simulink model "Biped_Model1"  (R2019a)
settings: Solver=VariableStepAuto  StartTime=0.0  StopTime=Time(end)  FixedStep=.001  EnableMultiTasking=on
PreLoadFcn:
  | YBT_HomeDir = pwd;
  | 
  | % Code to use copy within this repository
  | addpath([YBT_HomeDir filesep 'Libraries' filesep 'CFL_Libs']);
  | startup_Contact_Forces
  | 
  | cd(YBT_HomeDir)
  | addpath(YBT_HomeDir);
  | addpath([YBT_HomeDir filesep 'Libraries']);
  | addpath([YBT_HomeDir filesep 'Images']);
  | 
  | Robot_Parameters
model workspace: external: MATLAB File C:\Users\nozaripo\Desktop\BipedalWalking_Simulink_ModelnData\Robot_Parameters.m (data not in the file)
values from neighbouring files (symbols this model uses):
  ankle_servo_kd = 4    [Robot_Parameters.m]
  ankle_servo_ki = 0    [Robot_Parameters.m]
  ankle_servo_kp = 70    [Robot_Parameters.m]
  ankle_to_midLow = 19    [Robot_Parameters.m]
  contact_damping = 50    [Robot_Parameters.m]
  contact_point_radius = 0.005    [Robot_Parameters.m]
  contact_stiffness = 90311    [Robot_Parameters.m]
  deriv_filter_coeff = 50    [Robot_Parameters.m]
  foot_mass = 1    [Robot_Parameters.m]
  height_plane = 0.1    [Robot_Parameters.m]
  hip_servo_kd = 30    [Robot_Parameters.m]
  hip_servo_ki = 0    [Robot_Parameters.m]
  hip_servo_kp = 300    [Robot_Parameters.m]
  init = -joint_angles(1,:)    [Script_Data.m]
  init_vel = -vel(1,:)    [Script_Data.m]
  joint_angles = joint_angles(:,end:-1:1)    [Script_Data.m]
  joint_damping = 0    [Robot_Parameters.m]
  joint_stiffness = 0    [Robot_Parameters.m]
  knee_servo_kd = 30    [Robot_Parameters.m]
  knee_servo_ki = 0    [Robot_Parameters.m]
  knee_servo_kp = 150    [Robot_Parameters.m]
  knee_to_midUpp = 19    [Robot_Parameters.m]
  linear_contact_flag = 0    [Robot_Parameters.m]
  lower_leg_CM_offset = 2.55    [Robot_Parameters.m]
  lower_leg_mass = 2.87    [Robot_Parameters.m]
  max_torque_ank = 45    [Robot_Parameters.m]
  max_torque_hip = 25    [Robot_Parameters.m]
  max_torque_kn = 30    [Robot_Parameters.m]
  midLow_to_knee = 19    [Robot_Parameters.m]
  midUpp_to_hip = 19    [Robot_Parameters.m]
  motion_time_constant = 0.01    [Robot_Parameters.m]
  motor_constant = 0.01    [Robot_Parameters.m]
  motor_inertia = 0    [Robot_Parameters.m]
  mu_k = 0.5    [Robot_Parameters.m]
  mu_s = 0.8    [Robot_Parameters.m]
  mu_vth = 0.1    [Robot_Parameters.m]
  pen_exp = 1.5    [Robot_Parameters.m]
  plane_x = 3    [Robot_Parameters.m]
  plane_y = 0.3    [Robot_Parameters.m]
  split_belt = 0    [Script_Data.m]
  Time = (0:.01:.01*209)'    [Script_Data.m]
  torso_mass = 27.17    [Robot_Parameters.m]
  torso_to_hip = 11    [Robot_Parameters.m]
  upper_leg_CM_offset = 2.55    [Robot_Parameters.m]
  upper_leg_length = 38    [Robot_Parameters.m]
  upper_leg_mass = 4.7    [Robot_Parameters.m]
  V_treadmill = -1.0    (= -1)    [Script_Data.m]
  YBT_Par = struct    [Robot_Parameters.m]
undefined symbols (not defined in the file or in its folder): Extr_Data_LinkHoles, X, Y, Z
libraries: nesl_utility x197, sm_lib x144, fl_lib x42, simulink x20, ee_lib x18, Contact_Forces_Lib x16, Parts_Lib x10, Multibody_Multiphysics_Lib x6, simulink_extras x1
(part 4 of 11)

== system Biped_Model1/Robot/Robot Leg L/Box to Belt In Force1 ==
  In : Inport
  L_Fx : Scope
  L_Fz : Scope
  Sphere to Plane Force Enabled nz1 : Subsystem  AncestorBlock=Contact_Forces_Lib/3D/Sphere to Plane Force Enabled  mask(Sphere to Plane Force){sphere_rad=contact_point_radius, plane_lenx=plane_x, plane_leny=plane_y, plane_depth=height_plane/2, force_law=Linear, k_contact=contact_stiffness, b_contact=contact_damping, pen_full_damp_F=pen_full_damp_F_pla2pla, pen_exponent=pen_exponent_pla2pla, custom_param_1=1, custom_param_2=1, friction_law=Stick-Slip Continuous, mu_kinetic=mu_k, mu_static=mu_s, v_thr=mu_vth, vis_on=on, vis_opc_en=0, vis_len_plaBz=vis_len_plaLz, vis_clr=vis_clr, vis_opc=vis_opc}
      mask prompts: sphere_rad "Sphere Radius (m)"; plane_lenx "Plane Length x (m)"; plane_leny "Plane Length y (m)"; plane_depth "Plane Depth to Reference Frame (m)"; force_law "Force Law"; k_contact "Contact Stiffness (N/m)"; b_contact "Contact Damping (N/(m/s))"; pen_full_damp_F "Penetration for full damping (m)"; pen_exponent "Penetration exponent (>=1)"; custom_param_1 "Custom Parameter 1"; custom_param_2 "Custom Parameter 2"; friction_law "Friction Law"; mu_kinetic "Coefficient of Kinetic Friction"; mu_static "Coefficient of Static Friction"; v_thr "Velocity Threshold (m/s)"; vis_on "Visualize Contact Surfaces"; vis_opc_en "Visualize Opacity Enable"; vis_len_plaBz "Depth Plane Surface Element (Z-Axis) (m)"; vis_clr "Color of Surface Element (RGB)"; vis_opc "Opacity of Surface Element (0-1)"
      mask help:
      | This subsystem implements a contact force between a sphere and a plane.  The force is active above and below the plane.
      |
      | Frame connected to PlaB port:
      | 1. Located at midpoint of plane (x, y, and z).
      | 2. Z-axis is normal to the surfaces where force is active.
      |
      | Frame connected to the SphF port:
      | 1. Located at center of sphere.
      | 2. Orientation does not matter.
      |
      | Output signal is a bus with intermediate calculations and total force. Click Help for a diagram describing this force.
      mask init:
      | if strcmp(get_param(gcb,'force_law'),'Linear')
      |     set_param([gcb '/Forces/Force Law'],'OverrideUsingVariant','Linear');
      | elseif strcmp(get_param(gcb,'force_law'),'Nonlinear')
      |     set_param([gcb '/Forces/Force Law'],'OverrideUsingVariant','Nonlinear');
      | elseif strcmp(get_param(gcb,'force_law'),'Custom')
      |     set_param([gcb '/Forces/Force Law'],'OverrideUsingVariant','Custom');
      | end
      | 
      | if strcmp(get_param(gcb,'friction_law'),'None')
      |     set_param([gcb '/Forces/Ff/Friction Law'],'OverrideUsingVariant','None');
      | elseif strcmp(get_param(gcb,'friction_law'),'Stick-Slip Continuous')
      |     set_param([gcb '/Forces/Ff/Friction Law'],'OverrideUsingVariant','Stick_Slip_C');
      | end
      | 
      | if strcmp(get_param(gcb,'vis_on'),'on')
      |     vis_opc_en = 1;
      | elseif strcmp(get_param(gcb,'vis_on'),'off')
      |     vis_opc_en = 0;
      | end
      mask Help: web(which('Sphere_to_Plane_Contact.html'));
      mask TypeOptions force_law: Linear | Nonlinear | Custom
      mask Callback force_law:
      | %maskStr = get_param(gcb,'MaskValues');
      | maskObj = Simulink.Mask.get(gcb);
      | pfd_h = maskObj.getParameter('pen_full_damp_F');
      | pex_h = maskObj.getParameter('pen_exponent');
      | cc1_h = maskObj.getParameter('custom_param_1');
      | cc2_h = maskObj.getParameter('custom_param_2');
      | if strcmp(get_param(gcb,'force_law'),'Linear')
      |     pfd_h.Visible = 'off';
      |     pex_h.Visible = 'off';
      |     cc1_h.Visible = 'off';
      |     cc2_h.Visible = 'off';
      | %    set_param(gcb,'MaskVisibilities',{'on' 'on' 'on' 'on' 'on' 'off' 'off' 'off' 'off'});
      | %    set_param(gcb,'MaskVisibilities',{'on' 'on' 'on' 'on' 'on' 'off' 'off' 'off' 'off'});
      | elseif strcmp(get_param(gcb,'force_law'),'Nonlinear')
      |     pfd_h.Visible = 'on';
      |     pex_h.Visible = 'on';
      |     cc1_h.Visible = 'off';
      |     cc2_h.Visible = 'off';
      |     %set_param(gcb,'MaskVisibilities',{'on' 'on' 'on' 'on' 'on' 'on' 'on' 'off' 'off'});
      | elseif strcmp(get_param(gcb,'force_law'),'Custom')
      |     pfd_h.Visible = 'off';
      |     pex_h.Visible = 'off';
      |     cc1_h.Visible = 'on';
      |     cc2_h.Visible = 'on';
      |     %set_param(gcb,'MaskVisibilities',{'on' 'on' 'on' 'on' 'on' 'off' 'off' 'on' 'on'});
      | end
      | %clear maskObj
      | 
      | %maskObj = Simulink.Mask.get(gcb);
      | %if strcmp(get_param(gcb,'x'),'on')
      | %else
      | %    yh.Visible = 'off';
      | %end
      mask TypeOptions friction_law: None | Stick-Slip Continuous
      mask Callback friction_law:
      | maskObj = Simulink.Mask.get(gcb);
      | muk_h = maskObj.getParameter('mu_kinetic');
      | mus_h = maskObj.getParameter('mu_static');
      | vth_h = maskObj.getParameter('v_thr');
      | if strcmp(get_param(gcb,'friction_law'),'None')
      |     muk_h.Visible = 'off';
      |     mus_h.Visible = 'off';
      |     vth_h.Visible = 'off';
      | elseif strcmp(get_param(gcb,'friction_law'),'Stick-Slip Continuous')
      |     muk_h.Visible = 'on';
      |     mus_h.Visible = 'on';
      |     vth_h.Visible = 'on';
      | end
      | clear maskObj
      mask Callback vis_on:
      | maskObj = Simulink.Mask.get(gcb);
      | vis_clr_h = maskObj.getParameter('vis_clr');
      | vis_opc_h = maskObj.getParameter('vis_opc');
      | vis_len_plaBz_h = maskObj.getParameter('vis_len_plaBz');
      | if strcmp(get_param(gcb,'vis_on'),'off')
      |     vis_len_plaBz_h.Visible = 'off';
      |     vis_clr_h.Visible = 'off';
      |     vis_opc_h.Visible = 'off';
      | elseif strcmp(get_param(gcb,'vis_on'),'on')
      |     vis_len_plaBz_h.Visible = 'on';
      |     vis_clr_h.Visible = 'on';
      |     vis_opc_h.Visible = 'on';
      | end
      | clear maskObj vis_clr_h vis_opc_h
      | clear vis_len_plaBz_h
      mask DialogControl Dim_Cont Prompt: Dimensions
      mask DialogControl Con_Cont Prompt: Contact
      mask DialogControl Fri_Cont Prompt: Friction
      mask DialogControl Container9 Prompt: Visual
      mask Display: image('Sphere_to_Plane_Contact_Enabled_IMAGE.jpg');
  Sphere to Plane Force Enabled nz2 : Subsystem  AncestorBlock=Contact_Forces_Lib/3D/Sphere to Plane Force Enabled  mask(Sphere to Plane Force){sphere_rad=contact_point_radius, plane_lenx=plane_x, plane_leny=plane_y, plane_depth=height_plane/2, force_law=Linear, k_contact=contact_stiffness, b_contact=contact_damping, pen_full_damp_F=pen_full_damp_F_pla2pla, pen_exponent=pen_exponent_pla2pla, custom_param_1=1, custom_param_2=1, friction_law=Stick-Slip Continuous, mu_kinetic=mu_k, mu_static=mu_s, v_thr=mu_vth, vis_on=on, vis_opc_en=0, vis_len_plaBz=vis_len_plaLz, vis_clr=vis_clr, vis_opc=vis_opc}
      mask prompts: sphere_rad "Sphere Radius (m)"; plane_lenx "Plane Length x (m)"; plane_leny "Plane Length y (m)"; plane_depth "Plane Depth to Reference Frame (m)"; force_law "Force Law"; k_contact "Contact Stiffness (N/m)"; b_contact "Contact Damping (N/(m/s))"; pen_full_damp_F "Penetration for full damping (m)"; pen_exponent "Penetration exponent (>=1)"; custom_param_1 "Custom Parameter 1"; custom_param_2 "Custom Parameter 2"; friction_law "Friction Law"; mu_kinetic "Coefficient of Kinetic Friction"; mu_static "Coefficient of Static Friction"; v_thr "Velocity Threshold (m/s)"; vis_on "Visualize Contact Surfaces"; vis_opc_en "Visualize Opacity Enable"; vis_len_plaBz "Depth Plane Surface Element (Z-Axis) (m)"; vis_clr "Color of Surface Element (RGB)"; vis_opc "Opacity of Surface Element (0-1)"
      mask help:
      | This subsystem implements a contact force between a sphere and a plane.  The force is active above and below the plane.
      |
      | Frame connected to PlaB port:
      | 1. Located at midpoint of plane (x, y, and z).
      | 2. Z-axis is normal to the surfaces where force is active.
      |
      | Frame connected to the SphF port:
      | 1. Located at center of sphere.
      | 2. Orientation does not matter.
      |
      | Output signal is a bus with intermediate calculations and total force. Click Help for a diagram describing this force.
      mask init: same as Biped_Model1/Robot/Robot Leg L/Box to Belt In Force1/Sphere to Plane Force Enabled nz1
      mask Help: web(which('Sphere_to_Plane_Contact.html'));
      mask TypeOptions force_law: Linear | Nonlinear | Custom
      mask Callback force_law:
      | %maskStr = get_param(gcb,'MaskValues');
      | maskObj = Simulink.Mask.get(gcb);
      | pfd_h = maskObj.getParameter('pen_full_damp_F');
      | pex_h = maskObj.getParameter('pen_exponent');
      | cc1_h = maskObj.getParameter('custom_param_1');
      | cc2_h = maskObj.getParameter('custom_param_2');
      | if strcmp(get_param(gcb,'force_law'),'Linear')
      |     pfd_h.Visible = 'off';
      |     pex_h.Visible = 'off';
      |     cc1_h.Visible = 'off';
      |     cc2_h.Visible = 'off';
      | %    set_param(gcb,'MaskVisibilities',{'on' 'on' 'on' 'on' 'on' 'off' 'off' 'off' 'off'});
      | %    set_param(gcb,'MaskVisibilities',{'on' 'on' 'on' 'on' 'on' 'off' 'off' 'off' 'off'});
      | elseif strcmp(get_param(gcb,'force_law'),'Nonlinear')
      |     pfd_h.Visible = 'on';
      |     pex_h.Visible = 'on';
      |     cc1_h.Visible = 'off';
      |     cc2_h.Visible = 'off';
      |     %set_param(gcb,'MaskVisibilities',{'on' 'on' 'on' 'on' 'on' 'on' 'on' 'off' 'off'});
      | elseif strcmp(get_param(gcb,'force_law'),'Custom')
      |     pfd_h.Visible = 'off';
      |     pex_h.Visible = 'off';
      |     cc1_h.Visible = 'on';
      |     cc2_h.Visible = 'on';
      |     %set_param(gcb,'MaskVisibilities',{'on' 'on' 'on' 'on' 'on' 'off' 'off' 'on' 'on'});
      | end
      | %clear maskObj
      | 
      | %maskObj = Simulink.Mask.get(gcb);
      | %if strcmp(get_param(gcb,'x'),'on')
      | %else
      | %    yh.Visible = 'off';
      | %end
      mask TypeOptions friction_law: None | Stick-Slip Continuous
      mask Callback friction_law:
      | maskObj = Simulink.Mask.get(gcb);
      | muk_h = maskObj.getParameter('mu_kinetic');
      | mus_h = maskObj.getParameter('mu_static');
      | vth_h = maskObj.getParameter('v_thr');
      | if strcmp(get_param(gcb,'friction_law'),'None')
      |     muk_h.Visible = 'off';
      |     mus_h.Visible = 'off';
      |     vth_h.Visible = 'off';
      | elseif strcmp(get_param(gcb,'friction_law'),'Stick-Slip Continuous')
      |     muk_h.Visible = 'on';
      |     mus_h.Visible = 'on';
      |     vth_h.Visible = 'on';
      | end
      | clear maskObj
      mask Callback vis_on:
      | maskObj = Simulink.Mask.get(gcb);
      | vis_clr_h = maskObj.getParameter('vis_clr');
      | vis_opc_h = maskObj.getParameter('vis_opc');
      | vis_len_plaBz_h = maskObj.getParameter('vis_len_plaBz');
      | if strcmp(get_param(gcb,'vis_on'),'off')
      |     vis_len_plaBz_h.Visible = 'off';
      |     vis_clr_h.Visible = 'off';
      |     vis_opc_h.Visible = 'off';
      | elseif strcmp(get_param(gcb,'vis_on'),'on')
      |     vis_len_plaBz_h.Visible = 'on';
      |     vis_clr_h.Visible = 'on';
      |     vis_opc_h.Visible = 'on';
      | end
      | clear maskObj vis_clr_h vis_opc_h
      | clear vis_len_plaBz_h
      mask DialogControl Dim_Cont Prompt: Dimensions
      mask DialogControl Con_Cont Prompt: Contact
      mask DialogControl Fri_Cont Prompt: Friction
      mask DialogControl Container9 Prompt: Visual
      mask Display: image('Sphere_to_Plane_Contact_Enabled_IMAGE.jpg');
  Sum : Sum  Inputs=|++
  Sum1 : Sum  Inputs=|++
  FacF1 : PMIOPort  Side=Left
  FacF2 : PMIOPort  Port=2  Side=Left
  PlaB : PMIOPort  Port=3  Side=Right
  Out : Outport
  Out1 : Outport  Port=2
  "L_Fz " : Outport  Port=3  VectorParamsAs1DForOutWhenUnconnected=on
  "L_Fx " : Outport  Port=4  VectorParamsAs1DForOutWhenUnconnected=on
  wires:
  Sphere to Plane Force Enabled nz1/1(Out) -> Out/1
  Sphere to Plane Force Enabled nz2/1(Out) -> Out1/1
  In/1 -> Sphere to Plane Force Enabled nz2/1(In), Sphere to Plane Force Enabled nz1/1(In)
  Sum/1 -> L_Fz/1, "L_Fz "/1
  Sphere to Plane Force Enabled nz2/2(F_N_h) -> Sum/2
  Sphere to Plane Force Enabled nz1/2(F_N_t) -> Sum/1
  Sphere to Plane Force Enabled nz1/3(F_f_t) -> Sum1/1
  Sum1/1 -> L_Fx/1, "L_Fx "/1
  Sphere to Plane Force Enabled nz2/3(F_f_h) -> Sum1/2
  connections:
  PlaB/RConn1 -- Sphere to Plane Force Enabled nz1/RConn1 -- Sphere to Plane Force Enabled nz2/RConn1
  Sphere to Plane Force Enabled nz2/LConn1 -- FacF2/RConn1
  Sphere to Plane Force Enabled nz1/LConn1 -- FacF1/RConn1

== system Biped_Model1/Robot/Robot Leg L/Contact Force Logging1 ==
  m1 : Inport
  m2 : Inport  Port=2
  Add : Sum  Inputs=2
  Add1 : Sum  Inputs=2
  Bus Selector : BusSelector  OutputSignals=Normal Force,Friction Force
  Bus Selector1 : BusSelector  OutputSignals=Normal Force,Friction Force
  Math Function : Math  Commented=on  Operator=square  SaturateOnIntegerOverflow=on
  Sqrt : Sqrt  Commented=on  SaturateOnIntegerOverflow=on
  Sum of Elements : Sum  Commented=on  Inputs=+
  Fn : Outport
  Ff : Outport  Port=2
  Fn_h : Outport  Port=3
  wires:
  Add1/1 -> Ff/1  "Friction Force"
  Add/1 -> Fn/1  "Normal Force"
  Bus Selector1/2 -> Add1/2  "<Friction Force>"
  Bus Selector/2 -> Add1/1  "<Friction Force>"
  Bus Selector1/1 -> Fn_h/1, Add/2  "<Normal Force>"
  Bus Selector/1 -> Add/1  "<Normal Force>"
  m2/1 -> Bus Selector1/1
  m1/1 -> Bus Selector/1
  Sum of Elements/1 -> Sqrt/1
  Math Function/1 -> Sum of Elements/1

== system Biped_Model1/Robot/Robot Leg L/Create Bus ==
  vx : Inport
  Bus Creator : BusCreator  Inputs=3
  Enable : Constant
  vy : Constant  Value=0
  bus : Outport
  wires:
  Enable/1 -> Bus Creator/1  "Enable"
  vy/1 -> Bus Creator/3  "vy"
  vx/1 -> Bus Creator/2  "vx"
  Bus Creator/1 -> bus/1

== system Biped_Model1/Robot/Robot Leg L/Hip Joint ==
  note: 1) Add Subsystem or Model blocks as valid variant choices.
      | 2) You cannot connect blocks at this level. At simulation, connectivity is automatically
      | determined, based on the active variant and port name matching.
  qRef : Inport
  Motion : Subsystem  VariantControl=actuatorType == 1
  Motor : Subsystem  VariantControl=actuatorType == 3
  Torque : Subsystem  VariantControl=actuatorType == 2
  B : PMIOPort  Side=Left
  F : PMIOPort  Port=2  Side=Right
  meas : Outport

== system Biped_Model1/Robot/Robot Leg L/Knee Joint ==
  note: 1) Add Subsystem or Model blocks as valid variant choices.
      | 2) You cannot connect blocks at this level. At simulation, connectivity is automatically
      | determined, based on the active variant and port name matching.
  qRef : Inport
  Motion : Subsystem  VariantControl=actuatorType == 1
  Motor : Subsystem  VariantControl=actuatorType == 3
  Torque : Subsystem  VariantControl=actuatorType == 2
  B : PMIOPort  Side=Left
  F : PMIOPort  Port=2  Side=Right
  meas : Outport

== system Biped_Model1/Robot/Robot Leg L/Package Measurements1 ==
  Fn : Inport
  Ff : Inport  Port=2
  ankle : Inport  Port=3
  knee : Inport  Port=4
  hip : Inport  Port=5
  Bus Creator3 : BusCreator  Inputs=11
  Extract Measurements : Subsystem
  Extract Measurements1 : Subsystem
  Extract Measurements2 : Subsystem
  meas : Outport
  wires:
  Fn/1 -> Bus Creator3/1  "normal_force"
  Ff/1 -> Bus Creator3/2  "friction_force"
  Extract Measurements2/3(torque) -> Bus Creator3/8  "hip_torque"
  Extract Measurements2/1(angle) -> Bus Creator3/7  "hip_angle"
  Extract Measurements1/3(torque) -> Bus Creator3/6  "knee_torque"
  Extract Measurements1/1(angle) -> Bus Creator3/5  "knee_angle"
  hip/1 -> Extract Measurements2/1(meas)
  knee/1 -> Extract Measurements1/1(meas)
  Extract Measurements/3(torque) -> Bus Creator3/4  "ankle_torque"
  Extract Measurements/1(angle) -> Bus Creator3/3  "ankle_angle"
  ankle/1 -> Extract Measurements/1(meas)
  Bus Creator3/1 -> meas/1
  Extract Measurements/2(speed) -> Bus Creator3/9  "ankle_speed"
  Extract Measurements1/2(speed) -> Bus Creator3/10  "knee_speed"
  Extract Measurements2/2(speed) -> Bus Creator3/11  "hip_speed"

== system Biped_Model1/Robot/Robot Leg L/moving block ==
  In1 : Inport
  Clock : Clock
  Derivative : Derivative
  Derivative1 : Derivative
  Multiply : Product
  PS-Simulink Converter : nesl_utility/PS-Simulink Converter  PhysicalDomain=network_engine_domain  SubClassName=ps_output  LeftPortType=input  RightPortType=output  PseudoPeriodic=off  Frequencies=[]  Unit=1  AffineConversion=off
  Prismatic Joint : sm_lib/Joints/Prismatic Joint  SenseConstraintForce=off  SenseConstraintForceX=off  SenseConstraintForceY=off  SenseConstraintForceZ=off  SenseConstraintTorque=off  SenseConstraintTorqueX=off  SenseConstraintTorqueY=off  SenseConstraintTorqueZ=off  SenseTotalForce=off  SenseTotalForceX=off  SenseTotalForceY=off  SenseTotalForceZ=off  SenseTotalTorque=off  SenseTotalTorqueX=off  SenseTotalTorqueY=off  SenseTotalTorqueZ=off  CompositeWrenchDir=FollowerOnBase  CompositeWrenchFrame=BaseFrame  EquilibriumPosition=0  EquilibriumPositionUnits=m  SpringStiffness=0  SpringStiffnessUnits=N/m  DampingCoefficient=0  DampingCoefficientUnits=N/(m/s)  TorqueActuationMode=ComputedTorque  MotionActuationMode=InputMotion  SensePosition=on  SenseVelocity=off  SenseAcceleration=off  SenseTorqueForce=off  SenseLowerLimitTorqueForce=off  SenseUpperLimitTorqueForce=off  LowerLimitSpecify=off  LowerLimitBound=-1  LowerLimitBoundUnits=m  LowerLimitStiffness=1e6  LowerLimitStiffnessUnits=N/m  LowerLimitDamping=1e3  LowerLimitDampingUnits=N/(m/s)  LowerLimitTransitionRegionWidth=1e-4  LowerLimitTransitionRegionWidthUnits=m  UpperLimitSpecify=off  UpperLimitBound=1  UpperLimitBoundUnits=m  UpperLimitStiffness=1e6  UpperLimitStiffnessUnits=N/m  UpperLimitDamping=1e3  UpperLimitDampingUnits=N/(m/s)  UpperLimitTransitionRegionWidth=1e-4  UpperLimitTransitionRegionWidthUnits=m  PositionTargetSpecify=off  PositionTargetPriority=High  PositionTargetValue=0  PositionTargetValueUnits=m  VelocityTargetSpecify=off  VelocityTargetPriority=High  VelocityTargetValue=0  VelocityTargetValueUnits=m/s
  Rigid Transform : sm_lib/Frames and Transforms/Rigid Transform  TranslationMethod=Cartesian  TranslationStandardOffset=0  TranslationLengthUnit=m  TranslationStandardAxis=+Z  TranslationCartesianOffset=[3 -.045 0]  TranslationROffset=0  TranslationROffsetUnits=m  TranslationZOffset=0  TranslationZOffsetUnits=m  TranslationThetaOffset=0  TranslationThetaOffsetUnits=deg  RotationMethod=StandardAxis  RotationAngleUnits=deg  RotationStandardAxis=+Y  RotationAngle=90  RotationArbitraryAxis=[0 0 1]  FollAlignAxisA=+X  BaseAlignAxisA=+Y  FollAlignAxisB=+Y  BaseAlignAxisB=+Z  RotationSequenceAxes=FollowerAxes  RotationSequence=XYX  RotationSequenceAngles=[0 0 0]  RotationSequenceAnglesUnits=deg  RotationMatrix=[1 0 0; 0 1 0; 0 0 1]
  Scope1 : Scope
  Scope6 : Scope
  Simulink-PS Converter : nesl_utility/Simulink-PS Converter  PhysicalDomain=network_engine_domain  SubClassName=ps_input  LeftPortType=input  RightPortType=output  PseudoPeriodic=off  Frequencies=[]  NoiseDistribution=none  NoiseParameters=[]  Unit=m  AffineConversion=off  FilteringAndDerivatives=provide  SimscapeFilterOrder=2  InputFilterTimeConstant=0.001  UdotUserProvided=2
  Solid : sm_lib/Body Elements/Solid  InertiaType=CalculateFromGeometry  Mass=1  MassUnits=kg  CenterOfMass=[0 0 0]  CenterOfMassUnits=m  MomentsOfInertia=[1 1 1]  MomentsOfInertiaUnits=kg*m^2  ProductsOfInertia=[0 0 0]  ProductsOfInertiaUnits=kg*m^2  BasedOnType=Density  Density=.01  DensityUnits=kg/m^3  DoExposeReferenceFrame=on  SerializedFrames=<Frames/>  GraphicType=FromGeometry  MarkerShape=Sphere  MarkerSize=10  GraphicVisPropType=SimpleVisualProperties  GraphicDiffuseColor=[1.0 0.0 0.0]  GraphicSpecularColor=[0.5 0.5 0.5 1.0]  GraphicAmbientColor=[0.15 0.15 0.15 1.0]  GraphicEmissiveColor=[0.0 0.0 0.0 1.0]  GraphicShininess=75  GraphicOpacity=1.0  GeometryShape=Brick  RectangleSize=[1 1]  RectangleSizeUnits=m  BrickDimensions=[15 3 1]  BrickDimensionUnits=cm  CylinderRadius=1  CylinderRadiusUnits=m  CylinderLength=1  CylinderLengthUnits=m  SphereRadius=1  SphereRadiusUnits=m  EllipsoidRadii=[1 1 1]  EllipsoidRadiiUnits=m  ExtrusionCrossSection=[1 1; -1 1; -1 -1; 1 -1]  ExtrusionCrossSectionUnits=m  ExtrusionLength=1  ExtrusionLengthUnits=m  PolygonNumSides=3  PolygonOuterRadius=1  PolygonOuterRadiusUnits=m  ExtGeomFileType=STEP  ExtGeomFileUnits=m  RevolutionCrossSection=[1 1; 1 -1; 2 -1; 2 1]  RevolutionCrossSectionUnits=m  RevolutionExtent=Full  RevolutionAngle=180  RevolutionAngleUnits=deg
  Conn1 : PMIOPort  Side=Left
  wires:
  Multiply/1 -> Simulink-PS Converter/1, Derivative/1, Scope6/1
  Derivative/1 -> Simulink-PS Converter/2, Derivative1/1
  In1/1 -> Multiply/2
  Derivative1/1 -> Simulink-PS Converter/3
  Clock/1 -> Multiply/1
  PS-Simulink Converter/1 -> Scope1/1
  connections:
  PS-Simulink Converter/LConn1 -- Prismatic Joint/RConn2
  Simulink-PS Converter/RConn1 -- Prismatic Joint/LConn2
  Rigid Transform/RConn1 -- Prismatic Joint/LConn1
  Prismatic Joint/RConn1 -- Solid/RConn1
  Rigid Transform/LConn1 -- Conn1/RConn1

== system Biped_Model1/Robot/Robot Leg R/Ankle Joint ==
  note: 1) Add Subsystem or Model blocks as valid variant choices.
      | 2) You cannot connect blocks at this level. At simulation, connectivity is automatically
      | determined, based on the active variant and port name matching.
  qRef : Inport
  Motion : Subsystem  VariantControl=actuatorType == 1
  Motor : Subsystem  VariantControl=actuatorType == 3
  Torque : Subsystem  VariantControl=actuatorType == 2
  B : PMIOPort  Side=Left
  F : PMIOPort  Port=2  Side=Right
  meas : Outport

== system Biped_Model1/Robot/Robot Leg R/Belt ==
  Spd : Inport
  Gain : Gain  Gain=1/(belt_d/2*0.8)
  Integrator : Integrator
  Revolute Roller {1..5} (5 alike) : sm_lib/Joints/Revolute Joint  SenseConstraintForce=off  SenseConstraintForceX=off  SenseConstraintForceY=off  SenseConstraintForceZ=off  SenseConstraintTorque=off  SenseConstraintTorqueX=off  SenseConstraintTorqueY=off  SenseConstraintTorqueZ=off  SenseTotalForce=off  SenseTotalForceX=off  SenseTotalForceY=off  SenseTotalForceZ=off  SenseTotalTorque=off  SenseTotalTorqueX=off  SenseTotalTorqueY=off  SenseTotalTorqueZ=off  CompositeWrenchDir=FollowerOnBase  CompositeWrenchFrame=BaseFrame  EquilibriumPosition=0  EquilibriumPositionUnits=deg  SpringStiffness=0  SpringStiffnessUnits=N*m/deg  DampingCoefficient=0  DampingCoefficientUnits=N*m/(deg/s)  TorqueActuationMode=ComputedTorque  MotionActuationMode=InputMotion  SensePosition=off  SenseVelocity=off  SenseAcceleration=off  SenseTorqueForce=off  SenseLowerLimitTorqueForce=off  SenseUpperLimitTorqueForce=off  LowerLimitSpecify=off  LowerLimitBound=-90  LowerLimitBoundUnits=deg  LowerLimitStiffness=1e4  LowerLimitStiffnessUnits=N*m/deg  LowerLimitDamping=10  LowerLimitDampingUnits=N*m/(deg/s)  LowerLimitTransitionRegionWidth=0.1  LowerLimitTransitionRegionWidthUnits=deg  UpperLimitSpecify=off  UpperLimitBound=90  UpperLimitBoundUnits=deg  UpperLimitStiffness=1e4  UpperLimitStiffnessUnits=N*m/deg  UpperLimitDamping=10  UpperLimitDampingUnits=N*m/(deg/s)  UpperLimitTransitionRegionWidth=0.1  UpperLimitTransitionRegionWidthUnits=deg  PositionTargetSpecify=off  PositionTargetPriority=High  PositionTargetValue=0  PositionTargetValueUnits=deg  VelocityTargetSpecify=off  VelocityTargetPriority=High  VelocityTargetValue=0  VelocityTargetValueUnits=deg/s
  Roller {1..5} (5 alike) : Parts_Lib/Cylinder  Tag=CustomStyle  cyl_radius=belt_d/2*0.8  cyl_length=belt_w  cyl_density=1000  cyl_color=custom  cyl_opacity=1  cyl_color_custom=roller_clr  mark_radius=[0.75 0.5]  mark_len_factor=1.01  mark_angle=60  mark_color=black  mark_opacity=1
  Simulink-PS Converter : nesl_utility/Simulink-PS Converter  PhysicalDomain=network_engine_domain  SubClassName=ps_input  LeftPortType=input  RightPortType=output  PseudoPeriodic=off  Frequencies=[]  NoiseDistribution=none  NoiseParameters=[]  Unit=1  AffineConversion=off  FilteringAndDerivatives=filter  SimscapeFilterOrder=2  InputFilterTimeConstant=0.01  UdotUserProvided=1
  Solid : sm_lib/Body Elements/Solid  InertiaType=CalculateFromGeometry  Mass=1  MassUnits=kg  CenterOfMass=[0 0 0]  CenterOfMassUnits=m  MomentsOfInertia=[1 1 1]  MomentsOfInertiaUnits=kg*m^2  ProductsOfInertia=[0 0 0]  ProductsOfInertiaUnits=kg*m^2  BasedOnType=Density  Density=1000  DensityUnits=kg/(m^3)  DoExposeReferenceFrame=on  SerializedFrames=<Frames/>  GraphicType=FromGeometry  MarkerShape=Sphere  MarkerSize=10  GraphicVisPropType=SimpleVisualProperties  GraphicDiffuseColor=[0.2 0.2 0.2]  GraphicSpecularColor=[0.5 0.5 0.5 1.0]  GraphicAmbientColor=[0.15 0.15 0.15 1.0]  GraphicEmissiveColor=[0.0 0.0 0.0 1.0]  GraphicShininess=75  GraphicOpacity=1.0  GeometryShape=GeneralExtrusion  RectangleSize=[1 1]  RectangleSizeUnits=m  BrickDimensions=[1 1 1]  BrickDimensionUnits=m  CylinderRadius=1  CylinderRadiusUnits=m  CylinderLength=1  CylinderLengthUnits=m  SphereRadius=1  SphereRadiusUnits=m  EllipsoidRadii=[1 1 1]  EllipsoidRadiiUnits=m  ExtrusionCrossSection=Extr_Data_LinkHoles(belt_l,belt_d,0.8*belt_d/2,5)  ExtrusionCrossSectionUnits=m  ExtrusionLength=belt_w  ExtrusionLengthUnits=m  PolygonNumSides=3  PolygonOuterRadius=1  PolygonOuterRadiusUnits=m  ExtGeomFileType=STEP  ExtGeomFileUnits=m  RevolutionCrossSection=[1 1; 1 -1; 2 -1; 2 1]  RevolutionCrossSectionUnits=m  RevolutionExtent=Full  RevolutionAngle=180  RevolutionAngleUnits=deg
  Transform Contact Ref : sm_lib/Frames and Transforms/Rigid Transform  TranslationMethod=StandardAxis  TranslationStandardOffset=belt_w/2+.01  TranslationLengthUnit=m  TranslationStandardAxis=-Y  TranslationCartesianOffset=[0 0 0]  TranslationROffset=0  TranslationROffsetUnits=m  TranslationZOffset=0  TranslationZOffsetUnits=m  TranslationThetaOffset=0  TranslationThetaOffsetUnits=deg  RotationMethod=RotationSequence  RotationAngleUnits=deg  RotationStandardAxis=+Z  RotationAngle=0  RotationArbitraryAxis=[0 0 1]  FollAlignAxisA=+X  BaseAlignAxisA=+Y  FollAlignAxisB=+Y  BaseAlignAxisB=+Z  RotationSequenceAxes=FollowerAxes  RotationSequence=XYZ  RotationSequenceAngles=[-90 0 0]  RotationSequenceAnglesUnits=deg  RotationMatrix=[1 0 0; 0 1 0; 0 0 1]
  Transform Ramp Center : sm_lib/Frames and Transforms/Rigid Transform  TranslationMethod=StandardAxis  TranslationStandardOffset=belt_l/2  TranslationLengthUnit=m  TranslationStandardAxis=+X  TranslationCartesianOffset=[0 0 0]  TranslationROffset=0  TranslationROffsetUnits=m  TranslationZOffset=0  TranslationZOffsetUnits=m  TranslationThetaOffset=0  TranslationThetaOffsetUnits=deg  RotationMethod=None  RotationAngleUnits=deg  RotationStandardAxis=+Z  RotationAngle=0  RotationArbitraryAxis=[0 0 1]  FollAlignAxisA=+X  BaseAlignAxisA=+Y  FollAlignAxisB=+Y  BaseAlignAxisB=+Z  RotationSequenceAxes=FollowerAxes  RotationSequence=XYX  RotationSequenceAngles=[0 0 0]  RotationSequenceAnglesUnits=deg  RotationMatrix=[1 0 0; 0 1 0; 0 0 1]
  Transform Roller 1 : sm_lib/Frames and Transforms/Rigid Transform  TranslationMethod=StandardAxis  TranslationStandardOffset=belt_l/2  TranslationLengthUnit=m  TranslationStandardAxis=-X  TranslationCartesianOffset=[0 0 0]  TranslationROffset=0  TranslationROffsetUnits=m  TranslationZOffset=0  TranslationZOffsetUnits=m  TranslationThetaOffset=0  TranslationThetaOffsetUnits=deg  RotationMethod=None  RotationAngleUnits=deg  RotationStandardAxis=+Z  RotationAngle=0  RotationArbitraryAxis=[0 0 1]  FollAlignAxisA=+X  BaseAlignAxisA=+Y  FollAlignAxisB=+Y  BaseAlignAxisB=+Z  RotationSequenceAxes=FollowerAxes  RotationSequence=XYX  RotationSequenceAngles=[0 0 0]  RotationSequenceAnglesUnits=deg  RotationMatrix=[1 0 0; 0 1 0; 0 0 1]
  Transform Roller 2 : sm_lib/Frames and Transforms/Rigid Transform  TranslationMethod=StandardAxis  TranslationStandardOffset=belt_l/4  TranslationLengthUnit=m  TranslationStandardAxis=-X  TranslationCartesianOffset=[0 0 0]  TranslationROffset=0  TranslationROffsetUnits=m  TranslationZOffset=0  TranslationZOffsetUnits=m  TranslationThetaOffset=0  TranslationThetaOffsetUnits=deg  RotationMethod=None  RotationAngleUnits=deg  RotationStandardAxis=+Z  RotationAngle=0  RotationArbitraryAxis=[0 0 1]  FollAlignAxisA=+X  BaseAlignAxisA=+Y  FollAlignAxisB=+Y  BaseAlignAxisB=+Z  RotationSequenceAxes=FollowerAxes  RotationSequence=XYX  RotationSequenceAngles=[0 0 0]  RotationSequenceAnglesUnits=deg  RotationMatrix=[1 0 0; 0 1 0; 0 0 1]
  Transform Roller 4 : sm_lib/Frames and Transforms/Rigid Transform  TranslationMethod=StandardAxis  TranslationStandardOffset=belt_l/4  TranslationLengthUnit=m  TranslationStandardAxis=+X  TranslationCartesianOffset=[0 0 0]  TranslationROffset=0  TranslationROffsetUnits=m  TranslationZOffset=0  TranslationZOffsetUnits=m  TranslationThetaOffset=0  TranslationThetaOffsetUnits=deg  RotationMethod=None  RotationAngleUnits=deg  RotationStandardAxis=+Z  RotationAngle=0  RotationArbitraryAxis=[0 0 1]  FollAlignAxisA=+X  BaseAlignAxisA=+Y  FollAlignAxisB=+Y  BaseAlignAxisB=+Z  RotationSequenceAxes=FollowerAxes  RotationSequence=XYX  RotationSequenceAngles=[0 0 0]  RotationSequenceAnglesUnits=deg  RotationMatrix=[1 0 0; 0 1 0; 0 0 1]
  Transform Roller 5 : sm_lib/Frames and Transforms/Rigid Transform  TranslationMethod=StandardAxis  TranslationStandardOffset=belt_l/2  TranslationLengthUnit=m  TranslationStandardAxis=+X  TranslationCartesianOffset=[0 0 0]  TranslationROffset=0  TranslationROffsetUnits=m  TranslationZOffset=0  TranslationZOffsetUnits=m  TranslationThetaOffset=0  TranslationThetaOffsetUnits=deg  RotationMethod=None  RotationAngleUnits=deg  RotationStandardAxis=+Z  RotationAngle=0  RotationArbitraryAxis=[0 0 1]  FollAlignAxisA=+X  BaseAlignAxisA=+Y  FollAlignAxisB=+Y  BaseAlignAxisB=+Z  RotationSequenceAxes=FollowerAxes  RotationSequence=XYX  RotationSequenceAngles=[0 0 0]  RotationSequenceAnglesUnits=deg  RotationMatrix=[1 0 0; 0 1 0; 0 0 1]
  Ctr : PMIOPort  Side=Right
  End : PMIOPort  Port=2  Side=Left
  wires:
  Spd/1 -> Gain/1  "Belt speed"
  Gain/1 -> Integrator/1  "Roller speed"
  Integrator/1 -> Simulink-PS Converter/1  "Roller Angle"
  connections:
  Transform Contact Ref/LConn1 -- Ctr/RConn1
  Solid/RConn1 -- Revolute Roller 3/LConn1 -- Transform Roller 2/LConn1 -- Transform Roller 4/LConn1 -- Transform Roller 1/LConn1 -- Transform Roller 5/LConn1 -- Transform Ramp Center/RConn1 -- Transform Contact Ref/RConn1
  Transform Ramp Center/LConn1 -- End/RConn1
  Revolute Roller 1/RConn1 -- Roller 1/LConn1
  Transform Roller 2/RConn1 -- Revolute Roller 2/LConn1
  Revolute Roller 4/LConn1 -- Transform Roller 4/RConn1
  Revolute Roller 5/LConn1 -- Transform Roller 5/RConn1
  Transform Roller 1/RConn1 -- Revolute Roller 1/LConn1
  Roller 2/LConn1 -- Revolute Roller 2/RConn1
  Roller 3/LConn1 -- Revolute Roller 3/RConn1
  Roller 4/LConn1 -- Revolute Roller 4/RConn1
  Roller 5/LConn1 -- Revolute Roller 5/RConn1
  Simulink-PS Converter/RConn1 -- Revolute Roller 1/LConn2 -- Revolute Roller 2/LConn2 -- Revolute Roller 3/LConn2 -- Revolute Roller 4/LConn2 -- Revolute Roller 5/LConn2

== system Biped_Model1/Robot/Robot Leg R/Box to Belt In Force ==
  In : Inport
  "R_Fx  " : Scope
  R_Fz : Scope
  Sphere to Plane Force Enabled nz1 : Subsystem  AncestorBlock=Contact_Forces_Lib/3D/Sphere to Plane Force Enabled  mask(Sphere to Plane Force){sphere_rad=contact_point_radius, plane_lenx=plane_x, plane_leny=plane_y, plane_depth=height_plane/2, force_law=Linear, k_contact=contact_stiffness, b_contact=contact_damping, pen_full_damp_F=pen_full_damp_F_pla2pla, pen_exponent=pen_exponent_pla2pla, custom_param_1=1, custom_param_2=1, friction_law=Stick-Slip Continuous, mu_kinetic=mu_k, mu_static=mu_s, v_thr=mu_vth, vis_on=on, vis_opc_en=0, vis_len_plaBz=vis_len_plaLz, vis_clr=vis_clr, vis_opc=vis_opc}
      mask prompts: sphere_rad "Sphere Radius (m)"; plane_lenx "Plane Length x (m)"; plane_leny "Plane Length y (m)"; plane_depth "Plane Depth to Reference Frame (m)"; force_law "Force Law"; k_contact "Contact Stiffness (N/m)"; b_contact "Contact Damping (N/(m/s))"; pen_full_damp_F "Penetration for full damping (m)"; pen_exponent "Penetration exponent (>=1)"; custom_param_1 "Custom Parameter 1"; custom_param_2 "Custom Parameter 2"; friction_law "Friction Law"; mu_kinetic "Coefficient of Kinetic Friction"; mu_static "Coefficient of Static Friction"; v_thr "Velocity Threshold (m/s)"; vis_on "Visualize Contact Surfaces"; vis_opc_en "Visualize Opacity Enable"; vis_len_plaBz "Depth Plane Surface Element (Z-Axis) (m)"; vis_clr "Color of Surface Element (RGB)"; vis_opc "Opacity of Surface Element (0-1)"
      mask help:
      | This subsystem implements a contact force between a sphere and a plane.  The force is active above and below the plane.
      |
      | Frame connected to PlaB port:
      | 1. Located at midpoint of plane (x, y, and z).
      | 2. Z-axis is normal to the surfaces where force is active.
      |
      | Frame connected to the SphF port:
      | 1. Located at center of sphere.
      | 2. Orientation does not matter.
      |
      | Output signal is a bus with intermediate calculations and total force. Click Help for a diagram describing this force.
      mask init: same as Biped_Model1/Robot/Robot Leg L/Box to Belt In Force1/Sphere to Plane Force Enabled nz1
      mask Help: web(which('Sphere_to_Plane_Contact.html'));
      mask TypeOptions force_law: Linear | Nonlinear | Custom
      mask Callback force_law:
      | %maskStr = get_param(gcb,'MaskValues');
      | maskObj = Simulink.Mask.get(gcb);
      | pfd_h = maskObj.getParameter('pen_full_damp_F');
      | pex_h = maskObj.getParameter('pen_exponent');
      | cc1_h = maskObj.getParameter('custom_param_1');
      | cc2_h = maskObj.getParameter('custom_param_2');
      | if strcmp(get_param(gcb,'force_law'),'Linear')
      |     pfd_h.Visible = 'off';
      |     pex_h.Visible = 'off';
      |     cc1_h.Visible = 'off';
      |     cc2_h.Visible = 'off';
      | %    set_param(gcb,'MaskVisibilities',{'on' 'on' 'on' 'on' 'on' 'off' 'off' 'off' 'off'});
      | %    set_param(gcb,'MaskVisibilities',{'on' 'on' 'on' 'on' 'on' 'off' 'off' 'off' 'off'});
      | elseif strcmp(get_param(gcb,'force_law'),'Nonlinear')
      |     pfd_h.Visible = 'on';
      |     pex_h.Visible = 'on';
      |     cc1_h.Visible = 'off';
      |     cc2_h.Visible = 'off';
      |     %set_param(gcb,'MaskVisibilities',{'on' 'on' 'on' 'on' 'on' 'on' 'on' 'off' 'off'});
      | elseif strcmp(get_param(gcb,'force_law'),'Custom')
      |     pfd_h.Visible = 'off';
      |     pex_h.Visible = 'off';
      |     cc1_h.Visible = 'on';
      |     cc2_h.Visible = 'on';
      |     %set_param(gcb,'MaskVisibilities',{'on' 'on' 'on' 'on' 'on' 'off' 'off' 'on' 'on'});
      | end
      | %clear maskObj
      | 
      | %maskObj = Simulink.Mask.get(gcb);
      | %if strcmp(get_param(gcb,'x'),'on')
      | %else
      | %    yh.Visible = 'off';
      | %end
      mask TypeOptions friction_law: None | Stick-Slip Continuous
      mask Callback friction_law:
      | maskObj = Simulink.Mask.get(gcb);
      | muk_h = maskObj.getParameter('mu_kinetic');
      | mus_h = maskObj.getParameter('mu_static');
      | vth_h = maskObj.getParameter('v_thr');
      | if strcmp(get_param(gcb,'friction_law'),'None')
      |     muk_h.Visible = 'off';
      |     mus_h.Visible = 'off';
      |     vth_h.Visible = 'off';
      | elseif strcmp(get_param(gcb,'friction_law'),'Stick-Slip Continuous')
      |     muk_h.Visible = 'on';
      |     mus_h.Visible = 'on';
      |     vth_h.Visible = 'on';
      | end
      | clear maskObj
      mask Callback vis_on:
      | maskObj = Simulink.Mask.get(gcb);
      | vis_clr_h = maskObj.getParameter('vis_clr');
      | vis_opc_h = maskObj.getParameter('vis_opc');
      | vis_len_plaBz_h = maskObj.getParameter('vis_len_plaBz');
      | if strcmp(get_param(gcb,'vis_on'),'off')
      |     vis_len_plaBz_h.Visible = 'off';
      |     vis_clr_h.Visible = 'off';
      |     vis_opc_h.Visible = 'off';
      | elseif strcmp(get_param(gcb,'vis_on'),'on')
      |     vis_len_plaBz_h.Visible = 'on';
      |     vis_clr_h.Visible = 'on';
      |     vis_opc_h.Visible = 'on';
      | end
      | clear maskObj vis_clr_h vis_opc_h
      | clear vis_len_plaBz_h
      mask DialogControl Dim_Cont Prompt: Dimensions
      mask DialogControl Con_Cont Prompt: Contact
      mask DialogControl Fri_Cont Prompt: Friction
      mask DialogControl Container9 Prompt: Visual
      mask Display: image('Sphere_to_Plane_Contact_Enabled_IMAGE.jpg');
  Sphere to Plane Force Enabled nz2 : Subsystem  AncestorBlock=Contact_Forces_Lib/3D/Sphere to Plane Force Enabled  mask(Sphere to Plane Force){sphere_rad=contact_point_radius, plane_lenx=plane_x, plane_leny=plane_y, plane_depth=height_plane/2, force_law=Linear, k_contact=contact_stiffness, b_contact=contact_damping, pen_full_damp_F=pen_full_damp_F_pla2pla, pen_exponent=pen_exponent_pla2pla, custom_param_1=1, custom_param_2=1, friction_law=Stick-Slip Continuous, mu_kinetic=mu_k, mu_static=mu_s, v_thr=mu_vth, vis_on=on, vis_opc_en=0, vis_len_plaBz=vis_len_plaLz, vis_clr=vis_clr, vis_opc=vis_opc}
      mask prompts: sphere_rad "Sphere Radius (m)"; plane_lenx "Plane Length x (m)"; plane_leny "Plane Length y (m)"; plane_depth "Plane Depth to Reference Frame (m)"; force_law "Force Law"; k_contact "Contact Stiffness (N/m)"; b_contact "Contact Damping (N/(m/s))"; pen_full_damp_F "Penetration for full damping (m)"; pen_exponent "Penetration exponent (>=1)"; custom_param_1 "Custom Parameter 1"; custom_param_2 "Custom Parameter 2"; friction_law "Friction Law"; mu_kinetic "Coefficient of Kinetic Friction"; mu_static "Coefficient of Static Friction"; v_thr "Velocity Threshold (m/s)"; vis_on "Visualize Contact Surfaces"; vis_opc_en "Visualize Opacity Enable"; vis_len_plaBz "Depth Plane Surface Element (Z-Axis) (m)"; vis_clr "Color of Surface Element (RGB)"; vis_opc "Opacity of Surface Element (0-1)"
      mask help:
      | This subsystem implements a contact force between a sphere and a plane.  The force is active above and below the plane.
      |
      | Frame connected to PlaB port:
      | 1. Located at midpoint of plane (x, y, and z).
      | 2. Z-axis is normal to the surfaces where force is active.
      |
      | Frame connected to the SphF port:
      | 1. Located at center of sphere.
      | 2. Orientation does not matter.
      |
      | Output signal is a bus with intermediate calculations and total force. Click Help for a diagram describing this force.
      mask init: same as Biped_Model1/Robot/Robot Leg L/Box to Belt In Force1/Sphere to Plane Force Enabled nz1
      mask Help: web(which('Sphere_to_Plane_Contact.html'));
      mask TypeOptions force_law: Linear | Nonlinear | Custom
      mask Callback force_law:
      | %maskStr = get_param(gcb,'MaskValues');
      | maskObj = Simulink.Mask.get(gcb);
      | pfd_h = maskObj.getParameter('pen_full_damp_F');
      | pex_h = maskObj.getParameter('pen_exponent');
      | cc1_h = maskObj.getParameter('custom_param_1');
      | cc2_h = maskObj.getParameter('custom_param_2');
      | if strcmp(get_param(gcb,'force_law'),'Linear')
      |     pfd_h.Visible = 'off';
      |     pex_h.Visible = 'off';
      |     cc1_h.Visible = 'off';
      |     cc2_h.Visible = 'off';
      | %    set_param(gcb,'MaskVisibilities',{'on' 'on' 'on' 'on' 'on' 'off' 'off' 'off' 'off'});
      | %    set_param(gcb,'MaskVisibilities',{'on' 'on' 'on' 'on' 'on' 'off' 'off' 'off' 'off'});
      | elseif strcmp(get_param(gcb,'force_law'),'Nonlinear')
      |     pfd_h.Visible = 'on';
      |     pex_h.Visible = 'on';
      |     cc1_h.Visible = 'off';
      |     cc2_h.Visible = 'off';
      |     %set_param(gcb,'MaskVisibilities',{'on' 'on' 'on' 'on' 'on' 'on' 'on' 'off' 'off'});
      | elseif strcmp(get_param(gcb,'force_law'),'Custom')
      |     pfd_h.Visible = 'off';
      |     pex_h.Visible = 'off';
      |     cc1_h.Visible = 'on';
      |     cc2_h.Visible = 'on';
      |     %set_param(gcb,'MaskVisibilities',{'on' 'on' 'on' 'on' 'on' 'off' 'off' 'on' 'on'});
      | end
      | %clear maskObj
      | 
      | %maskObj = Simulink.Mask.get(gcb);
      | %if strcmp(get_param(gcb,'x'),'on')
      | %else
      | %    yh.Visible = 'off';
      | %end
      mask TypeOptions friction_law: None | Stick-Slip Continuous
      mask Callback friction_law:
      | maskObj = Simulink.Mask.get(gcb);
      | muk_h = maskObj.getParameter('mu_kinetic');
      | mus_h = maskObj.getParameter('mu_static');
      | vth_h = maskObj.getParameter('v_thr');
      | if strcmp(get_param(gcb,'friction_law'),'None')
      |     muk_h.Visible = 'off';
      |     mus_h.Visible = 'off';
      |     vth_h.Visible = 'off';
      | elseif strcmp(get_param(gcb,'friction_law'),'Stick-Slip Continuous')
      |     muk_h.Visible = 'on';
      |     mus_h.Visible = 'on';
      |     vth_h.Visible = 'on';
      | end
      | clear maskObj
      mask Callback vis_on:
      | maskObj = Simulink.Mask.get(gcb);
      | vis_clr_h = maskObj.getParameter('vis_clr');
      | vis_opc_h = maskObj.getParameter('vis_opc');
      | vis_len_plaBz_h = maskObj.getParameter('vis_len_plaBz');
      | if strcmp(get_param(gcb,'vis_on'),'off')
      |     vis_len_plaBz_h.Visible = 'off';
      |     vis_clr_h.Visible = 'off';
      |     vis_opc_h.Visible = 'off';
      | elseif strcmp(get_param(gcb,'vis_on'),'on')
      |     vis_len_plaBz_h.Visible = 'on';
      |     vis_clr_h.Visible = 'on';
      |     vis_opc_h.Visible = 'on';
      | end
      | clear maskObj vis_clr_h vis_opc_h
      | clear vis_len_plaBz_h
      mask DialogControl Dim_Cont Prompt: Dimensions
      mask DialogControl Con_Cont Prompt: Contact
      mask DialogControl Fri_Cont Prompt: Friction
      mask DialogControl Container9 Prompt: Visual
      mask Display: image('Sphere_to_Plane_Contact_Enabled_IMAGE.jpg');
  Sum : Sum  Inputs=|++
  Sum1 : Sum  Inputs=|++
  FacF1 : PMIOPort  Side=Left
  FacF2 : PMIOPort  Port=2  Side=Left
  PlaB : PMIOPort  Port=3  Side=Right
  Out : Outport
  Out1 : Outport  Port=2
  "R_Fz " : Outport  Port=3  VectorParamsAs1DForOutWhenUnconnected=on
  R_Fx : Outport  Port=4  VectorParamsAs1DForOutWhenUnconnected=on
  wires:
  Sphere to Plane Force Enabled nz1/1(Out) -> Out/1
  Sphere to Plane Force Enabled nz2/1(Out) -> Out1/1
  In/1 -> Sphere to Plane Force Enabled nz2/1(In), Sphere to Plane Force Enabled nz1/1(In)
  Sphere to Plane Force Enabled nz1/2(F_N_t) -> Sum/1
  Sphere to Plane Force Enabled nz2/2(F_N_h) -> Sum/2
  Sum/1 -> "R_Fz "/1, R_Fz/1
  Sphere to Plane Force Enabled nz1/3(F_f_t) -> Sum1/1
  Sum1/1 -> R_Fx/1, "R_Fx  "/1
  Sphere to Plane Force Enabled nz2/3(F_f_h) -> Sum1/2
  connections:
  PlaB/RConn1 -- Sphere to Plane Force Enabled nz2/RConn1 -- Sphere to Plane Force Enabled nz1/RConn1
  Sphere to Plane Force Enabled nz2/LConn1 -- FacF2/RConn1
  Sphere to Plane Force Enabled nz1/LConn1 -- FacF1/RConn1

== system Biped_Model1/Robot/Robot Leg R/Contact Force Logging ==
  m1 : Inport
  m2 : Inport  Port=2
  Add : Sum  Inputs=2
  Add1 : Sum  Inputs=2
  Bus Selector : BusSelector  OutputSignals=Normal Force,Friction Force
  Bus Selector1 : BusSelector  OutputSignals=Normal Force,Friction Force
  Math Function : Math  Commented=on  Operator=square  SaturateOnIntegerOverflow=on
  Sqrt : Sqrt  Commented=on  SaturateOnIntegerOverflow=on
  Sum of Elements : Sum  Commented=on  Inputs=+
  Fn : Outport
  Ff : Outport  Port=2
  Fn_h : Outport  Port=3
  wires:
  Add1/1 -> Ff/1  "Friction Force"
  Add/1 -> Fn/1  "Normal Force"
  Bus Selector1/2 -> Add1/2  "<Friction Force>"
  Bus Selector/2 -> Add1/1  "<Friction Force>"
  Bus Selector1/1 -> Fn_h/1, Add/2  "<Normal Force>"
  Bus Selector/1 -> Add/1  "<Normal Force>"
  m2/1 -> Bus Selector1/1
  m1/1 -> Bus Selector/1
  Sum of Elements/1 -> Sqrt/1
  Math Function/1 -> Sum of Elements/1

== system Biped_Model1/Robot/Robot Leg R/Create Bus ==
  vx : Inport
  Bus Creator : BusCreator  Inputs=3
  Enable : Constant
  vy : Constant  Value=0
  bus : Outport
  wires:
  Enable/1 -> Bus Creator/1  "Enable"
  vy/1 -> Bus Creator/3  "vy"
  vx/1 -> Bus Creator/2  "vx"
  Bus Creator/1 -> bus/1

== system Biped_Model1/Robot/Robot Leg R/Hip Joint ==
  note: 1) Add Subsystem or Model blocks as valid variant choices.
      | 2) You cannot connect blocks at this level. At simulation, connectivity is automatically
      | determined, based on the active variant and port name matching.
  qRef : Inport
  Motion : Subsystem  VariantControl=actuatorType == 1
  Motor : Subsystem  VariantControl=actuatorType == 3
  Torque : Subsystem  VariantControl=actuatorType == 2
  B : PMIOPort  Side=Left
  F : PMIOPort  Port=2  Side=Right
  meas : Outport

== system Biped_Model1/Robot/Robot Leg R/Knee Joint ==
  note: 1) Add Subsystem or Model blocks as valid variant choices.
      | 2) You cannot connect blocks at this level. At simulation, connectivity is automatically
      | determined, based on the active variant and port name matching.
  qRef : Inport
  Motion : Subsystem  VariantControl=actuatorType == 1
  Motor : Subsystem  VariantControl=actuatorType == 3
  Torque : Subsystem  VariantControl=actuatorType == 2
  B : PMIOPort  Side=Left
  F : PMIOPort  Port=2  Side=Right
  meas : Outport

== system Biped_Model1/Robot/Robot Leg R/Package Measurements ==
  Fn : Inport
  Ff : Inport  Port=2
  ankle : Inport  Port=3
  knee : Inport  Port=4
  hip : Inport  Port=5
  Bus Creator3 : BusCreator  Inputs=11
  Extract Measurements : Subsystem
  Extract Measurements1 : Subsystem
  Extract Measurements2 : Subsystem
  meas : Outport
  wires:
  Fn/1 -> Bus Creator3/1  "normal_force"
  Ff/1 -> Bus Creator3/2  "friction_force"
  Extract Measurements2/3(torque) -> Bus Creator3/8  "hip_torque"
  Extract Measurements2/1(angle) -> Bus Creator3/7  "hip_angle"
  Extract Measurements1/3(torque) -> Bus Creator3/6  "knee_torque"
  Extract Measurements1/1(angle) -> Bus Creator3/5  "knee_angle"
  hip/1 -> Extract Measurements2/1(meas)
  knee/1 -> Extract Measurements1/1(meas)
  Extract Measurements/3(torque) -> Bus Creator3/4  "ankle_torque"
  Extract Measurements/1(angle) -> Bus Creator3/3  "ankle_angle"
  ankle/1 -> Extract Measurements/1(meas)
  Bus Creator3/1 -> meas/1
  Extract Measurements/2(speed) -> Bus Creator3/9  "ankle_speed"
  Extract Measurements1/2(speed) -> Bus Creator3/10  "knee_speed"
  Extract Measurements2/2(speed) -> Bus Creator3/11  "hip_speed"
